simulink model "SILModelBlock"  (R2022b)
settings: Solver=FixedStepDiscrete  StartTime=0.0  StopTime=10  FixedStep=T  RelTol=1e-3
PostLoadFcn:
  | rtwdemo_overrides={'CodeProfilingInstrumentation','CodeProfilingSaveOptions','CodeExecutionProfiling','LaunchReport','PassReuseOutputArgsAs','ProdHWDeviceType','PortableWordSizes','ProdIntDivRoundTo','GenerateCodeMetricsReport'};
  | rtwconfiguredemo(gcs,'ERT',rtwdemo_overrides{:});
  | rtwdemo_cs=getActiveConfigSet(gcs);
  | setProp(rtwdemo_cs,'CustomSymbolStr','$R$N$M');
  | set_param(gcs,'dirty','off');
  | clear rtwdemo_overrides rtwdemo_cs
  | 
  | SILModelBlockData
values from neighbouring files (symbols this model uses):
  T = 0.1    [SILModelBlockData.m]
CloseFcn:
  | try, close_system('rtwdemo_pil2_counter',0), end
Description:
  | Processor-in-the-Loop Code Verification
settings Model: FPTRunName=Active  SILPILSystemUnderTest=refmodels  Creator=The MathWorks, Inc.  LastModifiedBy=The MathWorks, Inc.
settings SolverCC: AlgebraicLoopSolver=TrustRegion  MaxZcPerStep=1
settings DataIOCC: SaveFormat=StructureWithTime  SaveOutput=off  SaveTime=off  SignalLoggingName=logsOut
settings OptimizationCC: DefaultParameterBehavior=Inlined  UseDivisionForNetSlopeComputation=on  InlineInvariantSignals=on  EnhancedBackFolding=on  BooleansAsBitfields=on  PassReuseOutputArgsAs=Individual arguments  ExpressionDepthLimit=2147483647  StateBitsets=on  DataBitsets=on  ZeroExternalMemoryAtStartup=off  ZeroInternalMemoryAtStartup=off  NoFixptDivByZeroProtection=on  EfficientFloat2IntCast=on  SimCompilerOptimization=on  OptimizeBlockOrder=speed  DifferentSizesBufferReuse=on  EfficientTunableParamExpr=on
settings DebuggingCC: ReadBeforeWriteMsg=DisableAll  WriteAfterWriteMsg=DisableAll  WriteAfterReadMsg=DisableAll  CheckExecutionContextPreStartOutputMsg=on  ParameterTunabilityLossMsg=error  FcnCallInpInsideContextMsg=warning  UnconnectedInputMsg=warning  UnconnectedOutputMsg=warning  UnconnectedLineMsg=warning  UniqueDataStoreMsg=error  AllowSymbolicDim=off  ModelReferenceSymbolNameMessage=none  StateNameClashWarn=warning  StrictBusMsg=ErrorOnBusTreatedAsVector  SymbolicDimsDataTypeCodeGenerationDiagnostic=none  SFUnexpectedBacktrackingDiag=warning  SFNoUnconditionalDefaultTransitionDiag=warning  SFExecutionAtInitializationDiag=none  SFMachineParentedDataDiag=warning  ArithmeticOperatorsInVariantConditions=warning
settings HardwareCC: ProdBitPerPointer=32  ProdBitPerSizeT=32  ProdBitPerPtrDiffT=32  ProdLargestAtomicInteger=Long  ProdLargestAtomicFloat=Double  ProdWordSize=32  ProdHWDeviceType=ARM Compatible->ARM Cortex  TargetHWDeviceType=Generic->32-bit Embedded Processor
settings ModelReferenceCC: EnableRefExpFcnMdlSchedulingChecks=on  CheckModelReferenceTargetMessage=none  PropagateSignalLabelsOutOfModel=off
settings SFSimCC: SimUseLocalCustomCode=off  MATLABDynamicMemAlloc=off  CustomCodeUndefinedFunction=UseInterfaceOnly
settings RTWCC: Description=Embedded Coder  SystemTargetFile=ert.tlc  TLCOptions=-p0 -aWarnNonSaturatedBlocks=0  TemplateMakefile=ert_default_tmf  GenerateReport=on  RTWVerbose=off  RTWUseLocalCustomCode=off  IncludeHyperlinkInReport=on  PortableWordSizes=on  CodeExecutionProfiling=on  CodeProfilingSaveOptions=AllData  GenerateTraceInfo=on  GenerateTraceReport=on  GenerateTraceReportSl=on  GenerateTraceReportSf=on  GenerateTraceReportEml=on
settings CodeAppCC: ForceParamTrailComments=on  IgnoreCustomStorageClasses=off  OperatorAnnotations=on  SimulinkDataObjDesc=on  SFDataObjDesc=on  CustomSymbolStrGlobalVar=rt$N$M  CustomSymbolStrType=$N$M  CustomSymbolStrFcn=$N$M$F  CustomSymbolStrMacro=$N$M  InsertBlockDesc=on  InternalIdentifier=Classic
settings ERTTargetCC: UtilityFuncGeneration=Shared location  GenerateSampleERTMain=on  IncludeMdlTerminateFcn=off  CombineSignalStateStructs=on  SupportNonFinite=off  SupportComplex=off  InlinedParameterPlacement=NonHierarchical  ERTCustomFileTemplate=example_file_process.tlc  ERTFilePackagingFormat=CompactWithDataFile
settings ConfigComp: CovMetricSettings=dw  CovSaveCumulativeToWorkspaceVar=on  CovSaveSingleToWorkspaceVar=on  CovExternalEMLEnable=off  CovSFcnEnable=off

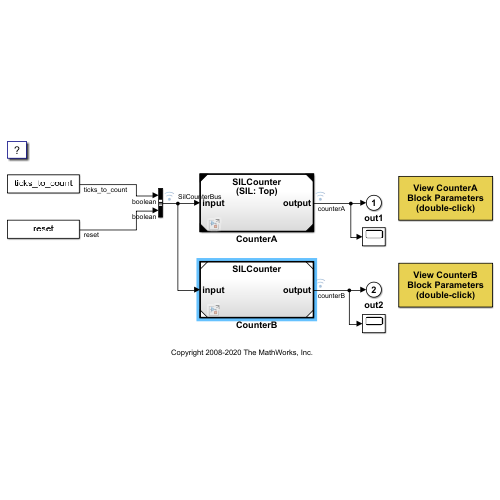
[thumbnail: Simulink's stored preview of the top-level diagram]
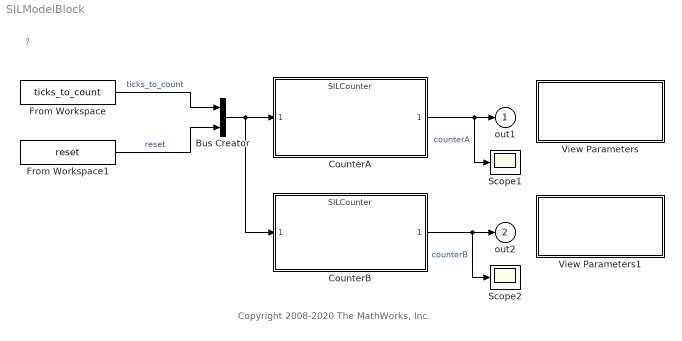
== system SILModelBlock ==
  note: Copyright 2008-2020 The MathWorks, Inc.
  note: ?
  Bus Creator : BusCreator  Inputs='ticks_to_count','reset'  OutDataTypeStr=Bus: SilCounterBus  NonVirtualBus=on
  CounterA : ModelReference  ModelNameDialog=SILCounter  SimulationMode=Software-in-the-loop (SIL)  CodeInterface=Top model  ModelReferenceVersion=6.2
  CounterB : ModelReference  ModelNameDialog=SILCounter  SimulationMode=Normal  ModelReferenceVersion=6.2
  From Workspace : FromWorkspace  VariableName=ticks_to_count  SampleTime=T
  From Workspace1 : FromWorkspace  VariableName=reset  SampleTime=T
  Scope1 : Scope
  Scope2 : Scope
  View Parameters : Subsystem
      settings: OpenFcn=|
      | hilite_system([bdroot '/CounterB'], 'none');
      | hilite_system([bdroot '/CounterA']);
      | open_system([bdroot '/CounterA'], 'parameter');
      mask Display: disp('View CounterA\nBlock Parameters\n(double-click)')
  View Parameters1 : Subsystem
      settings: OpenFcn=|
      | hilite_system([bdroot '/CounterA'], 'none');
      | hilite_system([bdroot '/CounterB']);
      | open_system([bdroot '/CounterB'], 'parameter');
      mask Display: disp('View CounterB\nBlock Parameters\n(double-click)')
  out1 : Outport  VectorParamsAs1DForOutWhenUnconnected=off
  out2 : Outport  Port=2  VectorParamsAs1DForOutWhenUnconnected=off
  wires:
  CounterA/1 -> out1/1, Scope1/1  "counterA"
  Bus Creator/1 -> CounterA/1, CounterB/1
  From Workspace/1 -> Bus Creator/1  "ticks_to_count"
  From Workspace1/1 -> Bus Creator/2  "reset"
  CounterB/1 -> out2/1, Scope2/1  "counterB"

== system SILModelBlock/View Parameters ==

== system SILModelBlock/View Parameters1 ==
